simulink model "motorcycle_model"  (Simulink 9.2)
settings: Solver=ode45  StartTime=0.0  StopTime=10.0  RelTol=1e-3  EnableMultiTasking=on
settings Model: Creator=W.Ooms  LastModifiedBy=Master Broda  SimulationMode=rapid-accelerator
settings DataIOCC: OutputOption=SpecifiedOutputTimes  OutputTimes=[0:0.05:10]
settings OptimizationCC: ExpressionDepthLimit=2147483647  InitFltsAndDblsToZero=on
settings DebuggingCC: SolverPrmCheckMsg=warning
settings SimscapeCC: SimscapeNormalizeSystem=off
settings ConfigurationSet: Description=SimMechanics 2G

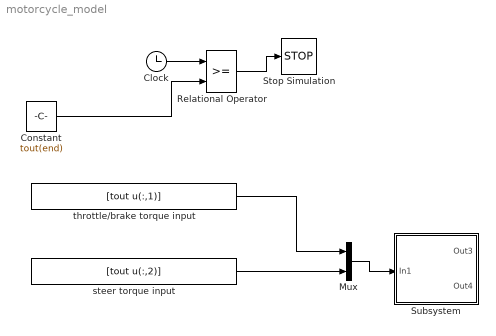
== system motorcycle_model ==
  Clock : Clock
  Constant : Constant  Value=tout(end)
  Mux : Mux  Inputs=2
  Relational Operator : RelationalOperator  OutDataTypeStr=boolean  RndMeth=Nearest
  Stop Simulation : Stop
  Subsystem : Subsystem
      mask init:
      | p=parameters('dummy');
      | q=coordinates('dummy');
      | pn = cell2mat(struct2cell(p));
  steer torque input : FromWorkspace  VariableName=[tout u(:,2)]  SampleTime=0  OutputAfterFinalValue=Holding final value
  throttle/brake torque input : FromWorkspace  VariableName=[tout u(:,1)]  SampleTime=0  OutputAfterFinalValue=Holding final value
  wires:
  steer torque input/1 -> Mux/2
  throttle/brake torque input/1 -> Mux/1
  Mux/1 -> Subsystem/1(In1)
  Clock/1 -> Relational Operator/1
  Relational Operator/1 -> Stop Simulation/1
  Constant/1 -> Relational Operator/2

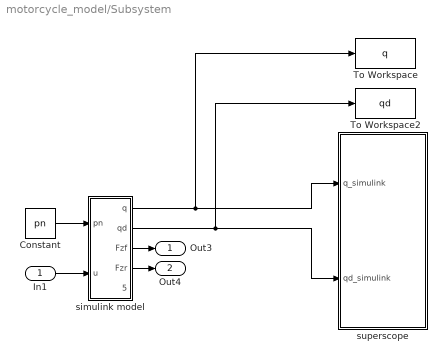
== system motorcycle_model/Subsystem ==
  In1 : Inport
  Constant : Constant  Value=pn
  To Workspace : ToWorkspace  VariableName=q  SampleTime=-1
  To Workspace2 : ToWorkspace  VariableName=qd  SampleTime=-1
  simulink model : Subsystem
  superscope : Subsystem
  Out3 : Outport
  Out4 : Outport  Port=2
  wires:
  simulink model/1(q) -> To Workspace/1, superscope/1(q_simulink)
  simulink model/2(qd) -> To Workspace2/1, superscope/2(qd_simulink)
  Constant/1 -> simulink model/1(pn)
  In1/1 -> simulink model/2(u)
  simulink model/3(Fzf) -> Out3/1
  simulink model/4(Fzr) -> Out4/1

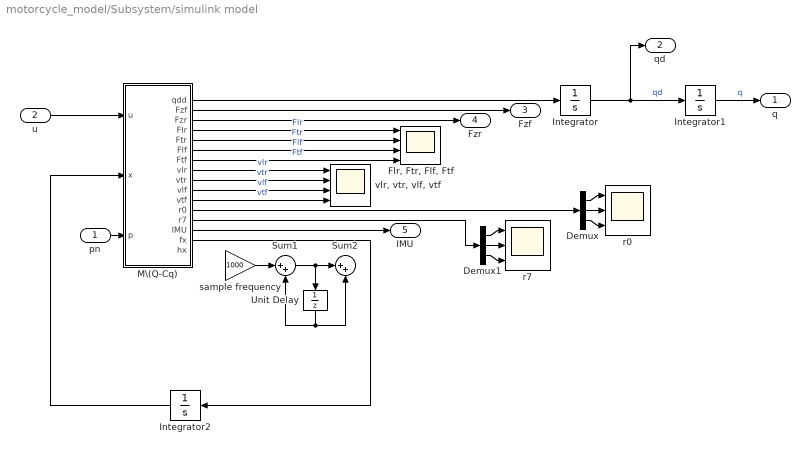
== system motorcycle_model/Subsystem/simulink model ==
  pn : Inport
  u : Inport  Port=2
  Demux : Demux  Outputs=3
  Demux1 : Demux  Outputs=3
  "Flr, Ftr, Flf, Ftf" : Scope  NumInputPorts=4
  Integrator : Integrator  InitialCondition=[q.qxd q.qyd q.qzd q.q0d q.q1d q.q2d q.q4d q.q5d q.q6d q.q7d q.qfd q.q8d q.q9d]
  Integrator1 : Integrator  InitialCondition=[q.qx q.qy q.qz q.q0 q.q1 q.q2 q.q4 q.q5 q.q6 q.q7 q.qf q.q8 q.q9]
  Integrator2 : Integrator  InitialCondition=[q.qxd q.qyd q.qzd q.q0d q.q1d q.q2d q.q4d q.q5d q.q6d q.q7d q.qfd q.q8d q.q9d q.qx q.qy q.qz q.q0 q.q1 q.q2 q.q4 q.q5 q.q6 q.q7 q.qf q.q8 q.q9]
  M\(Q-Cq) : MATLAB Function  TreatAsAtomicUnit=on
  Sum1 : Sum  Inputs=|++
  Sum2 : Sum  Inputs=|++
  Unit Delay : UnitDelay  InitialCondition=[q.qxd q.qyd q.qzd q.q0d q.q1d q.q2d q.q4d q.q5d q.q6d q.q7d q.qfd q.q8d q.q9d q.qx q.qy q.qz q.q0 q.q1 q.q2 q.q4 q.q5 q.q6 q.q7 q.qf q.q8 q.q9]  SampleTime=1/1000
  r0 : Scope  NumInputPorts=3
  r7 : Scope  NumInputPorts=3
  sample frequency : Gain  Gain=1000
  "vlr, vtr, vlf, vtf" : Scope  NumInputPorts=4
  q : Outport
  qd : Outport  Port=2
  Fzf : Outport  Port=3
  Fzr : Outport  Port=4
  IMU : Outport  Port=5
  wires:
  Integrator/1 -> Integrator1/1, qd/1  "qd"
  Integrator1/1 -> q/1  "q"
  M\(Q-Cq)/1(qdd) -> Integrator/1
  pn/1 -> M\(Q-Cq)/3(p)
  u/1 -> M\(Q-Cq)/1(u)
  M\(Q-Cq)/2(Fzf) -> Fzf/1
  M\(Q-Cq)/3(Fzr) -> Fzr/1
  M\(Q-Cq)/4(Flr) -> "Flr, Ftr, Flf, Ftf"/1  "Flr"
  M\(Q-Cq)/5(Ftr) -> "Flr, Ftr, Flf, Ftf"/2  "Ftr"
  M\(Q-Cq)/6(Flf) -> "Flr, Ftr, Flf, Ftf"/3  "Flf"
  M\(Q-Cq)/7(Ftf) -> "Flr, Ftr, Flf, Ftf"/4  "Ftf"
  M\(Q-Cq)/8(vlr) -> "vlr, vtr, vlf, vtf"/1  "vlr"
  M\(Q-Cq)/9(vtr) -> "vlr, vtr, vlf, vtf"/2  "vtr"
  M\(Q-Cq)/10(vlf) -> "vlr, vtr, vlf, vtf"/3  "vlf"
  M\(Q-Cq)/11(vtf) -> "vlr, vtr, vlf, vtf"/4  "vtf"
  Demux1/1 -> r7/1
  Demux1/2 -> r7/2
  Demux1/3 -> r7/3
  Demux/1 -> r0/1
  Demux/2 -> r0/2
  Demux/3 -> r0/3
  M\(Q-Cq)/12(r0) -> Demux/1
  M\(Q-Cq)/13(r7) -> Demux1/1
  M\(Q-Cq)/14(IMU) -> IMU/1
  M\(Q-Cq)/15(fx) -> Integrator2/1
  Sum1/1 -> Unit Delay/1, Sum2/1
  Unit Delay/1 -> Sum1/2, Sum2/2
  sample frequency/1 -> Sum1/1
  Integrator2/1 -> M\(Q-Cq)/2(x)

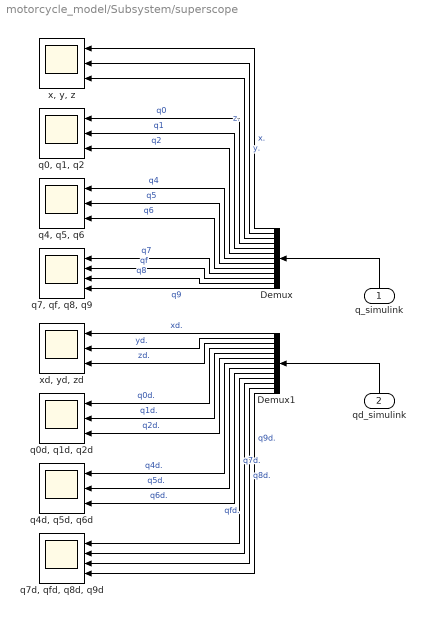
== system motorcycle_model/Subsystem/superscope ==
  q_simulink : Inport
  qd_simulink : Inport  Port=2
  Demux : Demux  Outputs=13
  Demux1 : Demux  Outputs=13
  "q0, q1, q2" : Scope  NumInputPorts=3
  "q0d, q1d, q2d" : Scope  NumInputPorts=3
  "q4, q5, q6" : Scope  NumInputPorts=3
  "q4d, q5d, q6d" : Scope  NumInputPorts=3
  "q7, qf, q8, q9" : Scope  NumInputPorts=4
  "q7d, qfd, q8d, q9d" : Scope  NumInputPorts=4
  "x, y, z" : Scope  NumInputPorts=3
  "xd, yd, zd" : Scope  NumInputPorts=3
  wires:
  q_simulink/1 -> Demux/1
  Demux/1 -> "x, y, z"/1  "x."
  Demux/2 -> "x, y, z"/2  "y."
  Demux/3 -> "x, y, z"/3  "z."
  Demux/4 -> "q0, q1, q2"/1  "q0"
  Demux/5 -> "q0, q1, q2"/2  "q1"
  Demux/6 -> "q0, q1, q2"/3  "q2"
  Demux/7 -> "q4, q5, q6"/1  "q4"
  Demux/8 -> "q4, q5, q6"/2  "q5"
  Demux/9 -> "q4, q5, q6"/3  "q6"
  Demux/10 -> "q7, qf, q8, q9"/1  "q7"
  Demux/11 -> "q7, qf, q8, q9"/2  "qf"
  Demux/12 -> "q7, qf, q8, q9"/3  "q8"
  Demux/13 -> "q7, qf, q8, q9"/4  "q9"
  qd_simulink/1 -> Demux1/1
  Demux1/1 -> "xd, yd, zd"/1  "xd."
  Demux1/2 -> "xd, yd, zd"/2  "yd."
  Demux1/3 -> "xd, yd, zd"/3  "zd."
  Demux1/4 -> "q0d, q1d, q2d"/1  "q0d."
  Demux1/5 -> "q0d, q1d, q2d"/2  "q1d."
  Demux1/6 -> "q0d, q1d, q2d"/3  "q2d."
  Demux1/7 -> "q4d, q5d, q6d"/1  "q4d."
  Demux1/8 -> "q4d, q5d, q6d"/2  "q5d."
  Demux1/9 -> "q4d, q5d, q6d"/3  "q6d."
  Demux1/10 -> "q7d, qfd, q8d, q9d"/1  "q7d."
  Demux1/11 -> "q7d, qfd, q8d, q9d"/2  "qfd."
  Demux1/12 -> "q7d, qfd, q8d, q9d"/3  "q8d."
  Demux1/13 -> "q7d, qfd, q8d, q9d"/4  "q9d."

== matlab function Subsystem/simulink model/M\(Q-Cq) ==
  data: u input double; qdd output double; x input double; p input double; Fzf output double; Fzr output double; Flr output double; Ftr output double; Flf output double; Ftf output double; vlr output double; vtr output double; vlf output double; vtf output double; r0 output double; r7 output double; IMU output double; fx output double; hx output double
function [qdd,Fzf,Fzr,Flr,Ftr,Flf,Ftf,vlr,vtr,vlf,vtf,r0,r7,IMU,fx,hx] = fcn(u,x,p)
[qdd,Fzf,Fzr,Flr,Ftr,Flf,Ftf,vlr,vtr,vlf,vtf,r0,r7,IMU,fx,hx]=mdl_motorcycle(u,x,p);
